simulink model "pmsm_controller_test_C_impl_r2009a"  (Simulink 7.6)
settings: Solver=FixedStepDiscrete  StartTime=0.0  StopTime=0.3  FixedStep=T_sim  RelTol=1e-3
InitFcn:
  | init_simulation
values from neighbouring files (symbols this model uses):
  C_Load = 0    [init_MIL.m]    (also in init_simulation.m)
  curr_adc_gain = 0.6247    [init_MIL.m]    (also in init_simulation.m)
  en_avr = 0    [init_MIL.m]    (also in init_simulation.m)
  FOC_CURR_GAIN_SCU10 = 640    [init_MIL.m]    (also in init_simulation.m)
  FOC_CURR_NULLIFICATION = 511    [init_MIL.m]    (also in init_simulation.m)
  FOC_K_FACTOR_FLUX_EST = 550    [init_simulation.m]
  FOC_SAMPLE_FREQ_HZ = 28000    [init_simulation.m]
  I_max = 106    [init_MIL.m]    (also in init_simulation.m = 100; plot_current_limits.m = 160)
  Id_ref_min = -1*160*0.8    (= -128)    [init_MIL.m]    (also in init_simulation.m)
  iq_set_fin_val = 100    [init_MIL.m]    (also in init_simulation.m)
  iq_set_init_val = 15    [init_MIL.m]    (also in init_simulation.m)
  iq_set_step_time = 0.005    [init_MIL.m]    (also in init_simulation.m)
  J_motor = (3.2220 + 11.438)*1e-6    (= 1.466e-05)    [init_MIL.m]    (also in init_simulation.m)
  Kpi = 0.3    [init_MIL.m]    (also in init_simulation.m)
  Kpi_n = 0.0015    [init_MIL.m]    (also in init_simulation.m)
  load_motor_spd_ramp = (load_motor_target_spd - load_motor_start_spd)/spd_ramp_time    (= 62831.8530718)    [init_MIL.m]    (also in init_simulation.m)
  load_motor_start_spd = 40000*2*pi/60    (= 4188.79020479)    [init_MIL.m]    (also in init_simulation.m)
  load_motor_target_spd = 70000*2*pi/60    (= 7330.38285838)    [init_MIL.m]    (also in init_simulation.m)
  Ls = 17.05e-6/3    (= 5.68333333333e-06)    [init_MIL.m]    (also in init_simulation.m; plot_current_limits.m)
  MOT_INDUCTANCE_SCU19 = 3    [init_simulation.m]
  MOT_RES_SCU19 = 2964    [init_simulation.m]
  N_avr = 1    [init_MIL.m]    (also in init_simulation.m)
  Nset_const = 50000    [init_MIL.m]    (also in init_simulation.m)
  ONEDIVSQRT3_SCU16 = 37837    [init_MIL.m]    (also in init_simulation.m)
  Pp = 1    [init_MIL.m]    (also in init_simulation.m; plot_current_limits.m)
  psi_p = 5.3e-3/sqrt(3)*0.95    [init_MIL.m]    (also in init_simulation.m)
  rate_i_falling = -100/0.02    (= -5000)    [init_MIL.m]    (also in init_simulation.m)
  rate_i_rising = 100/0.02    (= 5000)    [init_MIL.m]    (also in init_simulation.m)
  Rs = 10e-3*(1+0.0039*(120-20))/3    (= 0.00463333333333)    [init_MIL.m]    (also in init_simulation.m; plot_current_limits.m)
  Sel_Bench_Mode = 1    [init_MIL.m]    (also in init_simulation.m)
  Sel_Bench_Spd = 0    [init_MIL.m]    (also in init_simulation.m)
  Sel_id_ref = 2    [init_MIL.m]    (also in init_simulation.m)
  Sel_Iq_ref = 1    [init_MIL.m]    (also in init_simulation.m)
  Sel_Load = 1    [init_MIL.m]    (also in init_simulation.m)
  Set_Speed_rpm = 50000    [init_MIL.m]    (also in init_simulation.m)
  T_ctrl = T_pwm    (= 3.57002606119e-05)    [init_MIL.m]    (also in init_simulation.m)
  T_LUT_T = [0.1864, 0.1969, 0.2092, 0.2230, 0.2381, 0.2541, 0.2709, 0.2880, 0.3054, 0.3226, 0.3395, 0.3557, 0.3710, 0.3851, 0.3978, 0.4088, 0.4178 ... (first row only)    [init_MIL.m]    (also in init_simulation.m)
  T_pwm = 1/f_sw    (= 3.57002606119e-05)    [init_MIL.m]    (also in init_simulation.m)
  T_sim = T_pwm/100    (= 3.57002606119e-07)    [init_MIL.m]    (also in init_simulation.m)
  Tni = Ts    (= 0.00122661870504)    [init_MIL.m]    (also in init_simulation.m)
  Tni_n = Ts*1.5    (= 0.00183992805755)    [init_MIL.m]    (also in init_simulation.m)
  U_DC = V_dc    (= 36)    [init_simulation.m]
  V_dc = 36    [init_MIL.m]    (also in init_simulation.m)
libraries: simulink x32
(part 2 of 2)

== system pmsm_controller_test_C_impl_r2009a/FOC_Controller/VoltageRegulator/PI ==
  note: Manual Swich
      | Right Pos. Gain Scheduel
      | Left Pos. Constant Gain
  u_max : Inport
  u_amp : Inport  Port=2
  en : Inport  Port=3
  en_pi : Inport  Port=4
  Constant : Constant  Value=0
  Constant1 : Constant  Value=0
  Kpi_u : Gain  Gain=2^-4
  Kpi_u1 : Gain  Gain=2^-6
  SwI : Switch  Threshold=0.5
  Switch_I_Clr : Switch  Threshold=0.5
  Switch_PI : Switch  Threshold=0.5
  Unit Delay : UnitDelay  SampleTime=-1
  e_u_req : Sum  Inputs=+-
  int : Sum
  pi : Sum
  i_d : Outport
  wires:
  u_max/1 -> e_u_req/1
  Unit Delay/1 -> int/2
  pi/1 -> Switch_PI/1
  Switch_PI/1 -> i_d/1
  Kpi_u1/1 -> SwI/1
  en/1 -> SwI/3, SwI/2
  SwI/1 -> int/1
  int/1 -> pi/2, Switch_I_Clr/1
  Switch_I_Clr/1 -> Unit Delay/1
  e_u_req/1 -> Kpi_u1/1, Kpi_u/1
  u_amp/1 -> e_u_req/2
  en_pi/1 -> Switch_I_Clr/2, Switch_PI/2
  Constant/1 -> Switch_PI/3
  Constant1/1 -> Switch_I_Clr/3
  Kpi_u/1 -> pi/1

== system pmsm_controller_test_C_impl_r2009a/FOC_Controller/VoltageRegulator/SaturateIq ==
  CAN_I_max[A] : Inport
  Id_ref[A] : Inport  Port=2
  AntiDivByZero : Saturate  UpperLimit=inf  LowerLimit=1
  Divide : Product  Inputs=*/
  Product : Product  RndMeth=Zero
  acos : Trigonometry  Operator=acos
  sin : Trigonometry
  Iq_sat[A] : Outport
  wires:
  Id_ref[A]/1 -> Divide/1
  CAN_I_max[A]/1 -> AntiDivByZero/1
  AntiDivByZero/1 -> Divide/2, Product/2
  Divide/1 -> acos/1
  acos/1 -> sin/1
  sin/1 -> Product/1
  Product/1 -> Iq_sat[A]/1

== system pmsm_controller_test_C_impl_r2009a/IDEAL_VSI/Selector/If Action Subsystem ==
  In1 : Inport
  Action Port : ActionPort  PropagateVarSize=During execution  ActionType=then
  Out1 : Outport
  wires:
  In1/1 -> Out1/1

== system pmsm_controller_test_C_impl_r2009a/IDEAL_VSI/Selector/If Action Subsystem1 ==
  In1 : Inport
  Action Port : ActionPort  PropagateVarSize=During execution  ActionType=else
  Out1 : Outport
  wires:
  In1/1 -> Out1/1

== system pmsm_controller_test_C_impl_r2009a/IDEAL_VSI/Selector1/If Action Subsystem ==
  In1 : Inport
  Action Port : ActionPort  PropagateVarSize=During execution  ActionType=then
  Out1 : Outport
  wires:
  In1/1 -> Out1/1

== system pmsm_controller_test_C_impl_r2009a/IDEAL_VSI/Selector1/If Action Subsystem1 ==
  In1 : Inport
  Action Port : ActionPort  PropagateVarSize=During execution  ActionType=else
  Out1 : Outport
  wires:
  In1/1 -> Out1/1

== system pmsm_controller_test_C_impl_r2009a/IDEAL_VSI/Selector2/If Action Subsystem ==
  In1 : Inport
  Action Port : ActionPort  PropagateVarSize=During execution  ActionType=then
  Out1 : Outport
  wires:
  In1/1 -> Out1/1

== system pmsm_controller_test_C_impl_r2009a/IDEAL_VSI/Selector2/If Action Subsystem1 ==
  In1 : Inport
  Action Port : ActionPort  PropagateVarSize=During execution  ActionType=else
  Out1 : Outport
  wires:
  In1/1 -> Out1/1

== system pmsm_controller_test_C_impl_r2009a/IDEAL_VSI/Selector3/If Action Subsystem ==
  In1 : Inport
  Action Port : ActionPort  PropagateVarSize=During execution  ActionType=then
  Out1 : Outport
  wires:
  In1/1 -> Out1/1

== system pmsm_controller_test_C_impl_r2009a/IDEAL_VSI/Selector3/If Action Subsystem1 ==
  In1 : Inport
  Action Port : ActionPort  PropagateVarSize=During execution  ActionType=else
  Out1 : Outport
  wires:
  In1/1 -> Out1/1

== system pmsm_controller_test_C_impl_r2009a/IDEAL_VSI/Selector4/If Action Subsystem ==
  In1 : Inport
  Action Port : ActionPort  PropagateVarSize=During execution  ActionType=then
  Out1 : Outport
  wires:
  In1/1 -> Out1/1

== system pmsm_controller_test_C_impl_r2009a/IDEAL_VSI/Selector4/If Action Subsystem1 ==
  In1 : Inport
  Action Port : ActionPort  PropagateVarSize=During execution  ActionType=else
  Out1 : Outport
  wires:
  In1/1 -> Out1/1

== system pmsm_controller_test_C_impl_r2009a/IDEAL_VSI/Selector5/If Action Subsystem ==
  In1 : Inport
  Action Port : ActionPort  PropagateVarSize=During execution  ActionType=then
  Out1 : Outport
  wires:
  In1/1 -> Out1/1

== system pmsm_controller_test_C_impl_r2009a/IDEAL_VSI/Selector5/If Action Subsystem1 ==
  In1 : Inport
  Action Port : ActionPort  PropagateVarSize=During execution  ActionType=else
  Out1 : Outport
  wires:
  In1/1 -> Out1/1

== system pmsm_controller_test_C_impl_r2009a/PMSM/StatorEquation/Discrete_Integrator_al ==
  note: Unit delay is viewed equivalent to register in XSG
  In1 : Inport
  T_sample : Inport  Port=2
  Add : Sum  OutDataTypeStr=double
  Data Type Conversion : DataTypeConversion  OutDataTypeStr=double
  Data Type Conversion1 : DataTypeConversion  OutDataTypeStr=double
  Product : Product  OutDataTypeStr=double  RndMeth=Zero
  Unit Delay : UnitDelay  SampleTime=-1
  Out1 : Outport
  Out|z : Outport  Port=2
  wires:
  T_sample/1 -> Product/2
  Product/1 -> Add/1
  Unit Delay/1 -> Add/2, Data Type Conversion1/1
  Add/1 -> Unit Delay/1, Data Type Conversion/1
  In1/1 -> Product/1
  Data Type Conversion/1 -> Out1/1
  Data Type Conversion1/1 -> Out|z/1

== system pmsm_controller_test_C_impl_r2009a/PMSM/StatorEquation/Discrete_Integrator_be ==
  note: Unit delay is viewed equivalent to register in XSG
  In1 : Inport
  T_sample : Inport  Port=2
  Add : Sum  OutDataTypeStr=double
  Data Type Conversion : DataTypeConversion  OutDataTypeStr=double
  Data Type Conversion1 : DataTypeConversion  OutDataTypeStr=double
  Product : Product  OutDataTypeStr=double  RndMeth=Zero
  Unit Delay : UnitDelay  SampleTime=-1
  Out1 : Outport
  Out|z : Outport  Port=2
  wires:
  Data Type Conversion1/1 -> Out|z/1
  Data Type Conversion/1 -> Out1/1
  In1/1 -> Product/1
  Add/1 -> Data Type Conversion/1, Unit Delay/1
  Unit Delay/1 -> Data Type Conversion1/1, Add/2
  Product/1 -> Add/1
  T_sample/1 -> Product/2

== system pmsm_controller_test_C_impl_r2009a/PWM/SVPWM/SRF->3ph ==
  alpha beta : Inport  PortDimensions=2
  Mux : Mux  Inputs=3
  a : Fcn  Expr=u[1]
  b : Fcn  Expr=(-u[1]+sqrt(3)*u[2])/2
  c : Fcn  Expr=(-u[1]-sqrt(3)*u[2])/2
  abc : Outport
  wires:
  alpha beta/1 -> c/1, a/1, b/1
  Mux/1 -> abc/1
  c/1 -> Mux/3
  b/1 -> Mux/2
  a/1 -> Mux/1

== system pmsm_controller_test_C_impl_r2009a/PWM/ThreePhaseVoltageSource/dq-->alpha_beta2 ==
  eps : Inport
  u_q* : Inport  Port=2
  u_d* : Inport  Port=3
  Product{,1..3} (4 alike) : Product  RndMeth=Zero
  Sum2 : Sum  Inputs=|-+
  Sum3 : Sum  Inputs=|++
  Trigonometric Function : Trigonometry
  Trigonometric Function1 : Trigonometry  Operator=cos
  u_alpha* : Outport
  u_beta* : Outport  Port=2
  wires:
  Trigonometric Function/1 -> Product3/1, Product1/1
  Trigonometric Function1/1 -> Product/1, Product2/1
  u_q*/1 -> Product/2, Product1/2
  u_d*/1 -> Product3/2, Product2/2
  eps/1 -> Trigonometric Function/1, Trigonometric Function1/1
  Product1/1 -> Sum2/1
  Product2/1 -> Sum2/2
  Sum2/1 -> u_alpha*/1
  Product/1 -> Sum3/1
  Product3/1 -> Sum3/2
  Sum3/1 -> u_beta*/1

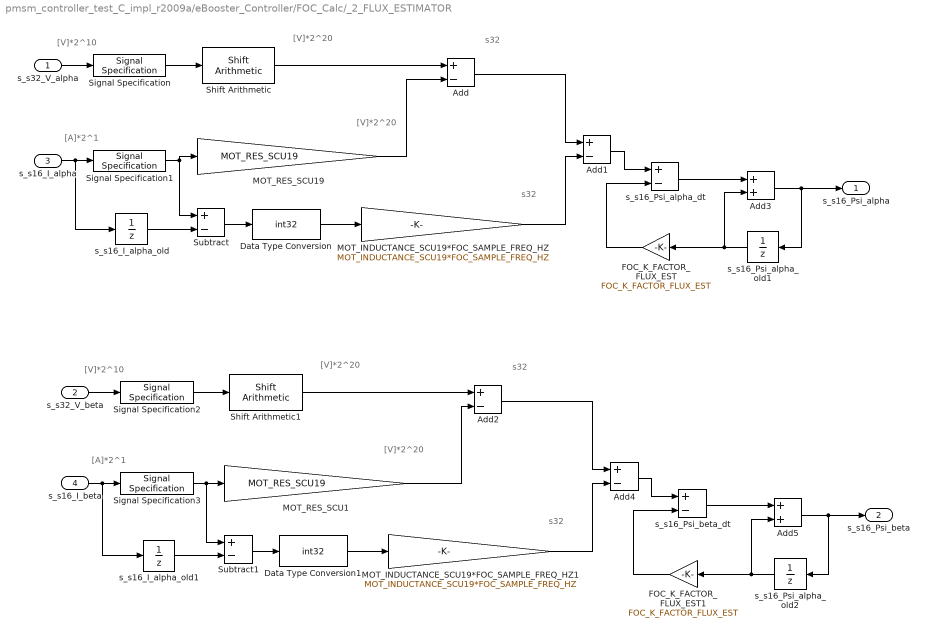
== system pmsm_controller_test_C_impl_r2009a/eBooster_Controller/FOC_Calc/_2_FLUX_ESTIMATOR ==
  note: [V]*2^10
  note: [A]*2^1
  note: [V]*2^20
  note: [V]*2^20
  note: s32
  note: s32
  note: [V]*2^10
  note: [A]*2^1
  note: [V]*2^20
  note: [V]*2^20
  note: s32
  note: s32
  s_s32_V_alpha : Inport
  s_s32_V_beta : Inport  Port=2
  s_s16_I_alpha : Inport  Port=3
  s_s16_I_beta : Inport  Port=4
  Add{,1..2,4} (4 alike) : Sum  Inputs=+-  AccumDataTypeStr=int32  OutDataTypeStr=int32
  Add3 : Sum  AccumDataTypeStr=int32  OutDataTypeStr=int32
  Add5 : Sum  AccumDataTypeStr=int32  OutDataTypeStr=int32
  Data Type Conversion : DataTypeConversion  OutDataTypeStr=int32
  Data Type Conversion1 : DataTypeConversion  OutDataTypeStr=int32
  FOC_K_FACTOR_FLUX_EST : Gain  Gain=FOC_K_FACTOR_FLUX_EST
  FOC_K_FACTOR_FLUX_EST1 : Gain  Gain=FOC_K_FACTOR_FLUX_EST
  MOT_INDUCTANCE_SCU19*FOC_SAMPLE_FREQ_HZ : Gain  Gain=MOT_INDUCTANCE_SCU19*FOC_SAMPLE_FREQ_HZ  ParamDataTypeStr=uint32  OutDataTypeStr=int32
  MOT_INDUCTANCE_SCU19*FOC_SAMPLE_FREQ_HZ1 : Gain  Gain=MOT_INDUCTANCE_SCU19*FOC_SAMPLE_FREQ_HZ  ParamDataTypeStr=uint32  OutDataTypeStr=int32
  MOT_RES_SCU1 : Gain  Gain=MOT_RES_SCU19  ParamDataTypeStr=uint16  OutDataTypeStr=int32
  MOT_RES_SCU19 : Gain  Gain=MOT_RES_SCU19  ParamDataTypeStr=uint16  OutDataTypeStr=int32
  Shift Arithmetic : simulink/Logic and Bit Operations/Shift Arithmetic  SystemSampleTime=-1  nBitShiftRight=-10  nBinPtShiftRight=0
  Shift Arithmetic1 : simulink/Logic and Bit Operations/Shift Arithmetic  SystemSampleTime=-1  nBitShiftRight=-10  nBinPtShiftRight=0
  Signal Specification : SignalSpecification  OutDataTypeStr=int32
  Signal Specification1 : SignalSpecification  OutDataTypeStr=int16
  Signal Specification2 : SignalSpecification  OutDataTypeStr=int32
  Signal Specification3 : SignalSpecification  OutDataTypeStr=int16
  Subtract : Sum  Inputs=+-
  Subtract1 : Sum  Inputs=+-
  s_s16_I_alpha_old : UnitDelay  SampleTime=-1
  s_s16_I_alpha_old1 : UnitDelay  SampleTime=-1
  s_s16_Psi_alpha_dt : Sum  Inputs=+-  AccumDataTypeStr=int32  OutDataTypeStr=int32
  s_s16_Psi_alpha_old1 : UnitDelay  SampleTime=-1
  s_s16_Psi_alpha_old2 : UnitDelay  SampleTime=-1
  s_s16_Psi_beta_dt : Sum  Inputs=+-  AccumDataTypeStr=int32  OutDataTypeStr=int32
  s_s16_Psi_alpha : Outport
  s_s16_Psi_beta : Outport  Port=2
  wires:
  s_s32_V_alpha/1 -> Signal Specification/1
  s_s16_I_alpha/1 -> Signal Specification1/1, s_s16_I_alpha_old/1
  Signal Specification/1 -> Shift Arithmetic/1
  Signal Specification1/1 -> MOT_RES_SCU19/1, Subtract/1
  Shift Arithmetic/1 -> Add/1
  MOT_RES_SCU19/1 -> Add/2
  Add/1 -> Add1/1
  s_s16_I_alpha_old/1 -> Subtract/2
  Subtract/1 -> Data Type Conversion/1
  Data Type Conversion/1 -> MOT_INDUCTANCE_SCU19*FOC_SAMPLE_FREQ_HZ/1
  MOT_INDUCTANCE_SCU19*FOC_SAMPLE_FREQ_HZ/1 -> Add1/2
  Add1/1 -> s_s16_Psi_alpha_dt/1
  FOC_K_FACTOR_FLUX_EST/1 -> s_s16_Psi_alpha_dt/2
  s_s16_Psi_alpha_dt/1 -> Add3/1
  Add3/1 -> s_s16_Psi_alpha_old1/1, s_s16_Psi_alpha/1
  s_s16_Psi_alpha_old1/1 -> Add3/2, FOC_K_FACTOR_FLUX_EST/1
  s_s32_V_beta/1 -> Signal Specification2/1
  s_s16_I_beta/1 -> s_s16_I_alpha_old1/1, Signal Specification3/1
  Signal Specification2/1 -> Shift Arithmetic1/1
  Signal Specification3/1 -> Subtract1/1, MOT_RES_SCU1/1
  Shift Arithmetic1/1 -> Add2/1
  MOT_RES_SCU1/1 -> Add2/2
  Add2/1 -> Add4/1
  s_s16_I_alpha_old1/1 -> Subtract1/2
  Subtract1/1 -> Data Type Conversion1/1
  Data Type Conversion1/1 -> MOT_INDUCTANCE_SCU19*FOC_SAMPLE_FREQ_HZ1/1
  MOT_INDUCTANCE_SCU19*FOC_SAMPLE_FREQ_HZ1/1 -> Add4/2
  Add4/1 -> s_s16_Psi_beta_dt/1
  FOC_K_FACTOR_FLUX_EST1/1 -> s_s16_Psi_beta_dt/2
  s_s16_Psi_beta_dt/1 -> Add5/1
  Add5/1 -> s_s16_Psi_alpha_old2/1, s_s16_Psi_beta/1
  s_s16_Psi_alpha_old2/1 -> FOC_K_FACTOR_FLUX_EST1/1, Add5/2

== system pmsm_controller_test_C_impl_r2009a/eBooster_Controller/MeasurementAndScaling/Iuvw_Meas ==
  note: -319A...319A
  note: Current scaling [A] --> digits
      | -319A...319A --> 0...1024
      | Note: Calibration not considered currently
  Iuvw[A] : Inport
  Bias : Bias  Bias=FOC_CURR_NULLIFICATION
  Data Type Conversion : DataTypeConversion  OutDataTypeStr=int16
  Gain : Gain  Gain=1/curr_adc_gain
  Saturation : Saturate  UpperLimit=319  LowerLimit=-319
  S16_Iuvw_ADC : Outport
  wires:
  Data Type Conversion/1 -> S16_Iuvw_ADC/1
  Bias/1 -> Data Type Conversion/1
  Gain/1 -> Bias/1
  Saturation/1 -> Gain/1
  Iuvw[A]/1 -> Saturation/1

== system pmsm_controller_test_C_impl_r2009a/eBooster_Controller/MeasurementAndScaling/_0_ADC_EVALUATION _1_CLARKE_TRANSFORMATION1 ==
  note: sint16
  note: W
  note: V
  note: U
  note: 1...6
  note: No FREEWHEELING and SYNC_CL States
  se_Sector : Inport
  i_uvw_adc : Inport  Port=2
  Demux : Demux  Outputs=3
  Merge : Merge  Inputs=3
  Merge1 : Merge  Inputs=3
  Mux1 : Mux  Inputs=2
  Mux2 : Mux  Inputs=2
  Mux3 : Mux  Inputs=2
  Switch Case : SwitchCase  CaseConditions={[1,6],[2,3],[4,5]}  ShowDefaultCase=off
  sector_1_6 : Subsystem  TreatAsAtomicUnit=on
  sector_2_3 : Subsystem  TreatAsAtomicUnit=on
  sector_4_5 : Subsystem  TreatAsAtomicUnit=on
  s_s16_I_alpha : Outport
  s_s16_I_beta : Outport  Port=2
  wires:
  Merge1/1 -> s_s16_I_beta/1
  sector_4_5/2(s_s16_I_beta) -> Merge1/3
  sector_2_3/2(s_s16_I_beta) -> Merge1/2
  sector_1_6/2(s_s16_I_beta) -> Merge1/1
  sector_4_5/1(s_s16_I_alpha) -> Merge/3
  sector_2_3/1(s_s16_I_alpha) -> Merge/2
  sector_1_6/1(s_s16_I_alpha) -> Merge/1
  Mux2/1 -> sector_4_5/1(In1)
  Demux/1 -> Mux2/1, Mux3/2
  Mux3/1 -> sector_2_3/1(In1)
  Demux/2 -> Mux2/2, Mux1/2
  Demux/3 -> Mux1/1, Mux3/1
  Mux1/1 -> sector_1_6/1(In1)
  Switch Case/3 -> sector_4_5/Action
  Switch Case/2 -> sector_2_3/Action
  Switch Case/1 -> sector_1_6/Action
  Merge/1 -> s_s16_I_alpha/1
  i_uvw_adc/1 -> Demux/1
  se_Sector/1 -> Switch Case/1

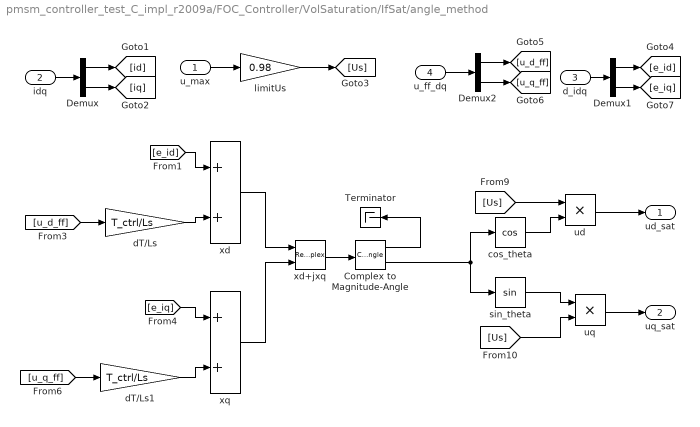
== system pmsm_controller_test_C_impl_r2009a/FOC_Controller/VolSaturation/IfSat/angle_method ==
  u_max : Inport
  idq : Inport  Port=2
  d_idq : Inport  Port=3
  u_ff_dq : Inport  Port=4
  Complex to Magnitude-Angle : ComplexToMagnitudeAngle
  Demux : Demux  Outputs=2
  Demux1 : Demux  Outputs=2
  Demux2 : Demux  Outputs=2
  Terminator : Terminator
  cos_theta : Trigonometry  Operator=cos
  dT/Ls : Gain  Gain=T_ctrl/Ls
  dT/Ls1 : Gain  Gain=T_ctrl/Ls
  limitUs : Gain  Gain=0.98
  sin_theta : Trigonometry
  ud : Product  RndMeth=Zero
  uq : Product  RndMeth=Zero
  xd : Sum
  xd+jxq : RealImagToComplex
  xq : Sum
  ud_sat : Outport
  uq_sat : Outport  Port=2
  wires:
  idq/1 -> Demux/1
  d_idq/1 -> Demux1/1
  Demux/1 -> [id]
  Demux/2 -> [iq]
  u_max/1 -> limitUs/1
  Complex to Magnitude-Angle/2 -> cos_theta/1, sin_theta/1
  [Us] -> ud/1
  cos_theta/1 -> ud/2
  sin_theta/1 -> uq/1
  [Us] -> uq/2
  Demux2/1 -> [u_d_ff]
  Demux2/2 -> [u_q_ff]
  u_ff_dq/1 -> Demux2/1
  Demux1/1 -> [e_id]
  Demux1/2 -> [e_iq]
  [e_id] -> xd/1
  dT/Ls/1 -> xd/2
  [u_d_ff] -> dT/Ls/1
  [e_iq] -> xq/1
  dT/Ls1/1 -> xq/2
  [u_q_ff] -> dT/Ls1/1
  xd/1 -> xd+jxq/1
  xq/1 -> xd+jxq/2
  xd+jxq/1 -> Complex to Magnitude-Angle/1
  Complex to Magnitude-Angle/1 -> Terminator/1
  ud/1 -> ud_sat/1
  uq/1 -> uq_sat/1
  limitUs/1 -> [Us]

== system pmsm_controller_test_C_impl_r2009a/FOC_Controller/VolSaturation/IfSat/d_priority ==
  udq : Inport
  u_max : Inport  Port=2
  Abs : Abs
  Demux : Demux  Outputs=2
  Gain : Gain  Gain=-1
  Product : Product  RndMeth=Zero
  Product1 : Product  RndMeth=Zero
  Product2 : Product  RndMeth=Zero
  Saturation Dynamic : simulink/Discontinuities/Saturation Dynamic  SystemSampleTime=-1  OutMin=[]  OutMax=[]  OutDataTypeStr=Inherit: Same as second input  OutDataType=fixdt(1, 16)  OutScaling=2^-10  DoSatur=off
  Sign : Signum
  Sqrt : Math  Operator=sqrt  SaturateOnIntegerOverflow=on
  Subtract : Sum  Inputs=-+
  ud_sat : Outport
  uq_sat : Outport  Port=2
  wires:
  u_max/1 -> Product1/1, Product1/2, Saturation Dynamic/1, Gain/1
  Product/1 -> Subtract/1
  Product1/1 -> Subtract/2
  Subtract/1 -> Abs/1
  Saturation Dynamic/1 -> Product/1, Product/2, ud_sat/1
  Gain/1 -> Saturation Dynamic/3
  Sqrt/1 -> Product2/1
  udq/1 -> Demux/1
  Demux/1 -> Saturation Dynamic/2
  Demux/2 -> Sign/1
  Sign/1 -> Product2/2
  Product2/1 -> uq_sat/1
  Abs/1 -> Sqrt/1

== system pmsm_controller_test_C_impl_r2009a/eBooster_Controller/MeasurementAndScaling/_0_ADC_EVALUATION _1_CLARKE_TRANSFORMATION1/sector_1_6 ==
  note: ADC1
  note: sint32
  note: s16_Curr_V
  note: s16_Curr_W
  note: [A]*2
  note: s16_Curr_U
  note: sint16
  note: sint16
  note: [A]*2
  note: sint16
  note: sint16
  note: sint16
  note: [A]*2
  note: ADC0
  note: ADC scaling see Iuvw_Meas:
      | -319A ... 319A -> 0 ... 1024 digits
  In1 : Inport
  Action Port : ActionPort  PropagateVarSize=During execution  ActionType=case
  Add : Sum  OutDataTypeStr=int16
  Add1 : Sum  AccumDataTypeStr=int32  OutDataTypeStr=int32
  Bias : Bias  Bias=-FOC_CURR_NULLIFICATION
  Bias1 : Bias  Bias=-FOC_CURR_NULLIFICATION
  Data Type Conversion : DataTypeConversion  OutDataTypeStr=int16
  Demux : Demux  Outputs=2
  Gain : Gain  Gain=FOC_CURR_GAIN_SCU10  ParamDataTypeStr=uint16  OutDataTypeStr=int32
  Gain2 : Gain  Gain=FOC_CURR_GAIN_SCU10  ParamDataTypeStr=uint16  OutDataTypeStr=int32
  Gain4 : Gain  Gain=ONEDIVSQRT3_SCU16  OutDataTypeStr=int32
  Gain6 : Gain  OutDataTypeStr=int16
  Gain7 : Gain  Gain=-1  ParamDataTypeStr=int32  OutDataTypeStr=int16
  Shift Arithmetic : simulink/Logic and Bit Operations/Shift Arithmetic  SystemSampleTime=-1  nBitShiftRight=9  nBinPtShiftRight=0
  Shift Arithmetic1 : simulink/Logic and Bit Operations/Shift Arithmetic  SystemSampleTime=-1  nBitShiftRight=9  nBinPtShiftRight=0
  Shift_l1 : simulink/Logic and Bit Operations/Shift Arithmetic  SystemSampleTime=-1  nBitShiftRight=-1  nBinPtShiftRight=0
  Shift_l16 : simulink/Logic and Bit Operations/Shift Arithmetic  SystemSampleTime=-1  nBitShiftRight=16  nBinPtShiftRight=0
  s_s16_I_alpha : Outport
  s_s16_I_beta : Outport  Port=2
  wires:
  Gain7/1 -> Shift_l1/1
  Shift_l16/1 -> Data Type Conversion/1
  Gain4/1 -> Shift_l16/1
  Add1/1 -> Gain4/1
  Shift_l1/1 -> Add1/2
  Add/1 -> Gain6/1, Add1/1
  Demux/2 -> Bias1/1
  Shift Arithmetic1/1 -> Gain7/1, Add/2
  Gain2/1 -> Shift Arithmetic1/1
  Bias1/1 -> Gain2/1
  Shift Arithmetic/1 -> Add/1
  Gain/1 -> Shift Arithmetic/1
  Bias/1 -> Gain/1
  Demux/1 -> Bias/1
  In1/1 -> Demux/1
  Gain6/1 -> s_s16_I_alpha/1
  Data Type Conversion/1 -> s_s16_I_beta/1

== system pmsm_controller_test_C_impl_r2009a/eBooster_Controller/MeasurementAndScaling/_0_ADC_EVALUATION _1_CLARKE_TRANSFORMATION1/sector_2_3 ==
  note: [A]*2
  note: s16_Curr_W
  note: s16_Curr_U
  note: s16_Curr_V
  note: sint32
  note: ADC0
  note: [A]*2
  note: sint16
  note: sint16
  note: sint16
  note: [A]*2
  note: sint16
  note: sint16
  note: ADC scaling see Iuvw_Meas:
      | -319A ... 319A -> 0 ... 1024 digits
  In1 : Inport
  Action Port : ActionPort  PropagateVarSize=During execution  ActionType=case
  Add : Sum  OutDataTypeStr=int16
  Add2 : Sum  AccumDataTypeStr=int32  OutDataTypeStr=int32
  Bias : Bias  Bias=-FOC_CURR_NULLIFICATION
  Bias1 : Bias  Bias=-FOC_CURR_NULLIFICATION
  Data Type Conversion : DataTypeConversion  OutDataTypeStr=int16
  Demux : Demux  Outputs=2
  Gain : Gain  Gain=FOC_CURR_GAIN_SCU10  OutDataTypeStr=int32
  Gain1 : Gain  Gain=-1  ParamDataTypeStr=int32  OutDataTypeStr=int16
  Gain2 : Gain  Gain=FOC_CURR_GAIN_SCU10  OutDataTypeStr=int32
  Gain3 : Gain  Gain=-1  ParamDataTypeStr=int32  OutDataTypeStr=int16
  Gain4 : Gain  Gain=ONEDIVSQRT3_SCU16  OutDataTypeStr=int32
  Gain5 : Gain  Gain=-1  ParamDataTypeStr=int32
  Gain6 : Gain  OutDataTypeStr=int16
  Shift Arithmetic : simulink/Logic and Bit Operations/Shift Arithmetic  SystemSampleTime=-1  nBitShiftRight=9  nBinPtShiftRight=0
  Shift Arithmetic1 : simulink/Logic and Bit Operations/Shift Arithmetic  SystemSampleTime=-1  nBitShiftRight=9  nBinPtShiftRight=0
  Shift_l1 : simulink/Logic and Bit Operations/Shift Arithmetic  SystemSampleTime=-1  nBitShiftRight=-1  nBinPtShiftRight=0
  Shift_l16 : simulink/Logic and Bit Operations/Shift Arithmetic  SystemSampleTime=-1  nBitShiftRight=16  nBinPtShiftRight=0
  s_s16_I_alpha : Outport
  s_s16_I_beta : Outport  Port=2
  wires:
  Gain6/1 -> s_s16_I_alpha/1
  Gain5/1 -> Shift_l1/1
  Data Type Conversion/1 -> s_s16_I_beta/1
  Add/1 -> Gain5/1
  Shift_l16/1 -> Data Type Conversion/1
  Gain4/1 -> Shift_l16/1
  Add2/1 -> Gain4/1
  Shift_l1/1 -> Add2/2
  In1/1 -> Demux/1
  Bias/1 -> Gain/1
  Gain/1 -> Shift Arithmetic/1
  Shift Arithmetic/1 -> Gain1/1
  Gain1/1 -> Gain6/1, Add2/1, Add/1
  Bias1/1 -> Gain2/1
  Gain2/1 -> Shift Arithmetic1/1
  Shift Arithmetic1/1 -> Gain3/1
  Gain3/1 -> Add/2
  Demux/1 -> Bias1/1
  Demux/2 -> Bias/1

== system pmsm_controller_test_C_impl_r2009a/eBooster_Controller/MeasurementAndScaling/_0_ADC_EVALUATION _1_CLARKE_TRANSFORMATION1/sector_4_5 ==
  note: sint16
  note: s16_Curr_U
  note: s16_Curr_V
  note: sint32
  note: sint16
  note: sint16
  note: [A]*2
  note: sint16
  note: sint16
  note: [A]*2
  note: ADC0
  note: ADC scaling see Iuvw_Meas:
      | -319A ... 319A -> 0 ... 1024 digits
  In1 : Inport
  Action Port : ActionPort  PropagateVarSize=During execution  ActionType=case
  Add2 : Sum  AccumDataTypeStr=int32  OutDataTypeStr=int32
  Bias : Bias  Bias=-FOC_CURR_NULLIFICATION
  Bias1 : Bias  Bias=-FOC_CURR_NULLIFICATION
  Data Type Conversion : DataTypeConversion  OutDataTypeStr=int16
  Demux : Demux  Outputs=2
  Gain : Gain  Gain=FOC_CURR_GAIN_SCU10  OutDataTypeStr=int32
  Gain1 : Gain  Gain=-1  ParamDataTypeStr=int32  OutDataTypeStr=int16
  Gain2 : Gain  Gain=FOC_CURR_GAIN_SCU10  OutDataTypeStr=int32
  Gain3 : Gain  Gain=-1  ParamDataTypeStr=int32  OutDataTypeStr=int16
  Gain4 : Gain  Gain=ONEDIVSQRT3_SCU16  OutDataTypeStr=int32
  Gain6 : Gain  OutDataTypeStr=int16
  Shift Arithmetic : simulink/Logic and Bit Operations/Shift Arithmetic  SystemSampleTime=-1  nBitShiftRight=9  nBinPtShiftRight=0
  Shift Arithmetic1 : simulink/Logic and Bit Operations/Shift Arithmetic  SystemSampleTime=-1  nBitShiftRight=9  nBinPtShiftRight=0
  Shift_l1 : simulink/Logic and Bit Operations/Shift Arithmetic  SystemSampleTime=-1  nBitShiftRight=-1  nBinPtShiftRight=0
  Shift_l16 : simulink/Logic and Bit Operations/Shift Arithmetic  SystemSampleTime=-1  nBitShiftRight=16  nBinPtShiftRight=0
  s_s16_I_alpha : Outport
  s_s16_I_beta : Outport  Port=2
  wires:
  Gain6/1 -> s_s16_I_alpha/1
  Data Type Conversion/1 -> s_s16_I_beta/1
  Shift_l16/1 -> Data Type Conversion/1
  Gain4/1 -> Shift_l16/1
  Add2/1 -> Gain4/1
  Shift_l1/1 -> Add2/2
  Gain3/1 -> Shift_l1/1
  Demux/2 -> Bias1/1
  Shift Arithmetic1/1 -> Gain3/1
  Gain2/1 -> Shift Arithmetic1/1
  Bias1/1 -> Gain2/1
  Gain1/1 -> Gain6/1, Add2/1
  Shift Arithmetic/1 -> Gain1/1
  Gain/1 -> Shift Arithmetic/1
  Bias/1 -> Gain/1
  Demux/1 -> Bias/1
  In1/1 -> Demux/1
